simulink model "DiscretizedPlant"  (R2022b)
settings: Solver=VariableStepAuto  StartTime=0.0  StopTime=10.0  RelTol=1e-3
undefined symbols (not defined in the file): den, num
settings Model: Creator=emanuelevitetta  LastModifiedBy=emanuelevitetta

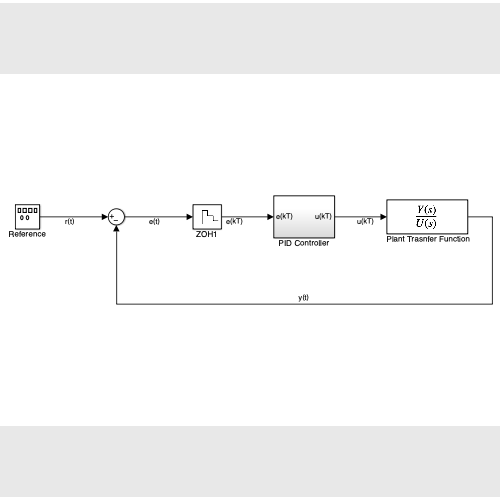
[thumbnail: Simulink's stored preview of the top-level diagram]
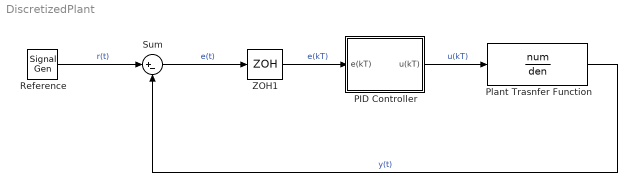
== system DiscretizedPlant ==
  " Plant Trasnfer Function" : TransferFcn  Numerator=num  Denominator=den
  PID Controller : Subsystem
  Reference : SignalGenerator  Units=rad/sec
  Sum : Sum  Inputs=|+-
  ZOH1 : ZeroOrderHold  SampleTime=-1
  wires:
  PID Controller/1(u(kT)) -> " Plant Trasnfer Function"/1  "u(kT)"
  Reference/1 -> Sum/1  "r(t)"
  Sum/1 -> ZOH1/1  "e(t)"
  " Plant Trasnfer Function"/1 -> Sum/2  "y(t)"
  ZOH1/1 -> PID Controller/1(e(kT))  "e(kT)"

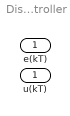
== system DiscretizedPlant/PID Controller ==
  e(kT) : Inport
  u(kT) : Outport
